simulink model "BMS_Software_NXP_Rolo"  (R2020a)
settings: Solver=FixedStepDiscrete  StartTime=0.0  StopTime=10.0  FixedStep=0.05  RelTol=1e-3  EnableMultiTasking=on
InitFcn:
  | mbd_s32k_consistency_checks(bdroot(gcs));
undefined symbols (not defined in the file or in its folder): LQFP
libraries: mbd_bcc_ec_toolbox x51, mbd_s32k1xx_ec_toolbox x16
(part 1 of 3)
Description:
  | This model demonstrates how to use Model-Based Design Toolbox for S32K to run a BMS Algorithm, already validated in Matlab&Simulink environment.
  | This BMS Algorithm is available for free  on the Mathworks File Exchangehttps://www.mathworks.com/matlabcentral/fileexchange/72865-design-and-test-lithium-ion-battery-management-algorithms
  | 
  | Validation:
  | Hardware required: S32K144EVB + FRDM33772BSPIEVB + BATT-6EMULATOR
  | Once the model has been succesfully build it is automatically deployed on the target.
  | Open the BMS_Software_NXP.pmpx FreeMaster project, connect to the board and simulate the Algorithm states using the Cell Emulator.
settings Model: DataDictionary=BMS_Software_DD_NXP.sldd  EnableAccessToBaseWorkspace=off  PauseTimes=0  ExtModeTrigDuration=5  Creator=Chirag Patel  LastModifiedBy=RolandoA
settings SolverCC: AutoInsertRateTranBlk=on
settings DataIOCC: ExternalInput=off  InitialState=off  SaveOutput=off  SignalLogging=off  SaveTime=off
settings OptimizationCC: DefaultParameterBehavior=Inlined  EnhancedBackFolding=on  PassReuseOutputArgsAs=Individual arguments  ZeroExternalMemoryAtStartup=off  ZeroInternalMemoryAtStartup=off  OptimizeBlockOrder=speed  DifferentSizesBufferReuse=on  OptimizationCustomize=off  EfficientTunableParamExpr=on
settings DebuggingCC: UnderspecifiedInitializationDetection=Classic  MergeDetectMultiDrivingBlocksExec=none  InheritedTsInSrcMsg=none  SingleTaskRateTransMsg=error  ParameterPrecisionLossMsg=none  ParameterTunabilityLossMsg=error  UnconnectedInputMsg=error  UnconnectedOutputMsg=error  UnconnectedLineMsg=error  UnknownTsInhSupMsg=error
settings HardwareCC: ProdBitPerPointer=32  ProdBitPerSizeT=32  ProdBitPerPtrDiffT=32  ProdLargestAtomicInteger=Long  ProdLargestAtomicFloat=Double  ProdWordSize=32  ProdHWDeviceType=ARM Compatible->ARM Cortex
settings ModelReferenceCC: ModelReferenceNumInstancesAllowed=Single  PropagateSignalLabelsOutOfModel=off
settings SFSimCC: MATLABDynamicMemAlloc=off
settings RTWCC: Description=Model Based Design Toolbox S32K1xx Code Generation Target  SystemTargetFile=mbd_s32k.tlc  MakeCommand=mbd_s32k_make_rtw COPY_MDLREF_INCLUDES=0  TemplateMakefile=mbd_s32k.tmf  GenerateReport=on  IncludeHyperlinkInReport=on  LaunchReport=on  GenerateTraceInfo=on  GenerateTraceReport=on  GenerateTraceReportSl=on  GenerateTraceReportSf=on  GenerateTraceReportEml=on
settings CodeAppCC: ForceParamTrailComments=on  IgnoreCustomStorageClasses=off  OperatorAnnotations=on  SimulinkDataObjDesc=on  SFDataObjDesc=on  InsertBlockDesc=on
settings STFCustomTargetCC: TargetLangStandard=C99 (ISO)  MultiwordLength=256  CombineOutputUpdateFcns=on  ERTCustomFileBanners=on  SupportContinuousTime=off  SupportNonInlinedSFcns=off  RemoveResetFunc=on  MATLABClassNameForMDSCustomization=Simulink.SoftwareTarget.ERTCustomization  SystemTargetFile=mbd_s32k.tlc
settings ERTTargetCC: TargetLangStandard=C99 (ISO)  ParMdlRefBuildCompliant=off  CompOptLevelCompliant=off  ConcurrentExecutionCompliant=off  ModelStepFunctionPrototypeControlCompliant=off  CPPClassGenCompliant=off  UseToolchainInfoCompliant=off  InlinedParameterPlacement=NonHierarchical  ERTSrcFileBannerTemplate=mbd_ert_code_template.cgt  ERTHdrFileBannerTemplate=mbd_ert_code_template.cgt  ERTDataSrcFileTemplate=mbd_ert_code_template.cgt  ERTDataHdrFileTemplate=mbd_ert_code_template.cgt  ERTCustomFileTemplate=example_file_process.tlc

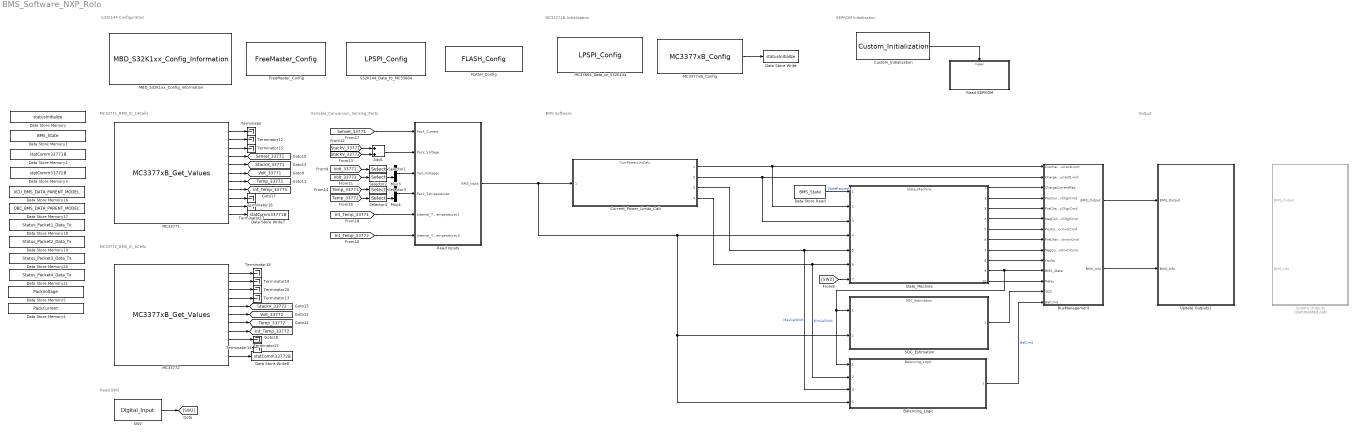
== system BMS_Software_NXP_Rolo ==
  note: EEPROM Initialization
  note: Read SW2
  note: MC33772B Initialization
  note: BMS Software
  note: S32K144 Configuration
  note: Output
  note: MC33771_BMS_IC_14Cells
  note: MC33772_BMS_IC_6Cells
  note: Variable_Conversion_Sensing_Parts
  Add1 : Sum  AccumDataTypeStr=single  OutDataTypeStr=single
  Balancing_Logic : ModelReference  ModelNameDialog=Balancing_Logic  SimulationMode=Normal  ModelReferenceVersion=1.581
      mask Display: image('Balancing.jpg',[70,5,200,90])
  BusManagement : Subsystem
  Current_Power_Limits_Calc : ModelReference  ModelNameDialog=CurrPowerLimCalc.slx  SimulationMode=Normal  ModelReferenceVersion=1.557
      mask Display: image('CurrentPowerLimit.png',[68,15,80,80])
  Custom_Initialization : mbd_s32k1xx_ec_toolbox/Utility Blocks/Custom_Initialization
  Data Store Memory : DataStoreMemory  DataStoreName=statusInitialize  ReadBeforeWriteMsg=warning  WriteAfterWriteMsg=warning  WriteAfterReadMsg=warning  ShowAdditionalParam=off
  Data Store Memory1 : DataStoreMemory  DataStoreName=BMS_State  ReadBeforeWriteMsg=warning  WriteAfterWriteMsg=warning  WriteAfterReadMsg=warning  InitialValue=SRE.Balancing  ShowAdditionalParam=off  OutDataTypeStr=Enum: SRE
  Data Store Memory16 : DataStoreMemory  DataStoreName=VCU_BMS_DATA_PARENT_MODEL  ReadBeforeWriteMsg=warning  WriteAfterWriteMsg=warning  WriteAfterReadMsg=warning  ShowAdditionalParam=off  OutDataTypeStr=Bus: VCU_BMS_DATA
  Data Store Memory17 : DataStoreMemory  DataStoreName=OBC_BMS_DATA_PARENT_MODEL  ReadBeforeWriteMsg=warning  WriteAfterWriteMsg=warning  WriteAfterReadMsg=warning  ShowAdditionalParam=off  OutDataTypeStr=Bus: OBC_BMS_DATA
  Data Store Memory18 : DataStoreMemory  DataStoreName=Status_Packet1_Data_Tx  ReadBeforeWriteMsg=warning  WriteAfterWriteMsg=warning  WriteAfterReadMsg=warning  ShowAdditionalParam=off  OutDataTypeStr=Bus: Status_Packet1_Data_Tx
  Data Store Memory19 : DataStoreMemory  DataStoreName=Status_Packet2_Data_Tx  ReadBeforeWriteMsg=warning  WriteAfterWriteMsg=warning  WriteAfterReadMsg=warning  ShowAdditionalParam=off  OutDataTypeStr=Bus: Status_Packet2_Data_Tx
  Data Store Memory2 : DataStoreMemory  DataStoreName=statComm33771B  ReadBeforeWriteMsg=warning  WriteAfterWriteMsg=warning  WriteAfterReadMsg=warning  ShowAdditionalParam=off
  Data Store Memory20 : DataStoreMemory  DataStoreName=Status_Packet3_Data_Tx  ReadBeforeWriteMsg=warning  WriteAfterWriteMsg=warning  WriteAfterReadMsg=warning  ShowAdditionalParam=off  OutDataTypeStr=Bus: Status_Packet3_Data_Tx
  Data Store Memory21 : DataStoreMemory  DataStoreName=Status_Packet4_Data_Tx  ReadBeforeWriteMsg=warning  WriteAfterWriteMsg=warning  WriteAfterReadMsg=warning  ShowAdditionalParam=off  OutDataTypeStr=Bus: Status_Packet4_Data_Tx
  Data Store Memory3 : DataStoreMemory  DataStoreName=statComm33772B  ReadBeforeWriteMsg=warning  WriteAfterWriteMsg=warning  WriteAfterReadMsg=warning  ShowAdditionalParam=off
  Data Store Memory4 : DataStoreMemory  DataStoreName=PackCurrent  ReadBeforeWriteMsg=warning  WriteAfterWriteMsg=warning  WriteAfterReadMsg=warning  ShowAdditionalParam=off  OutDataTypeStr=single
  Data Store Memory5 : DataStoreMemory  DataStoreName=PackVoltage  ReadBeforeWriteMsg=warning  WriteAfterWriteMsg=warning  WriteAfterReadMsg=warning  ShowAdditionalParam=off  OutDataTypeStr=single
  Data Store Read : DataStoreRead  DataStoreName=BMS_State
  Data Store Write : DataStoreWrite  DataStoreName=statusInitialize
  Data Store Write7 : DataStoreWrite  DataStoreName=statComm33771B
  Data Store Write8 : DataStoreWrite  DataStoreName=statComm33772B
  FLASH_Config : mbd_s32k1xx_ec_toolbox/Core and System Blocks/FLASH Blocks/FLASH_Config  depart=0x2  eeesize=4096  csec_en=off  csec_num_user_keys=5 keys
  FreeMaster_Config : mbd_s32k1xx_ec_toolbox/Utility Blocks/FreeMaster_Config  interface=LPUART2  baudrate=115200  rxd=PTD6: [LPUART2_RX | Receive]  txd=PTD7: [LPUART2_TX | Transmit]  mode=Short Interrupt  isr_prio=1  show_adv_opts=on  use_scope=on  max_scope_vars=8  use_recorder=off  max_rec_vars=8  rec_buff_size=1024  rec_timebase=0 milliseconds  comm_buffer_size_auto=on  comm_buffer_size=255  comm_rqueue_size_default=on  comm_rqueue_size=32
  MBD_S32K1xx_Config_Information : mbd_s32k1xx_ec_toolbox/MBD_S32K1xx_Config_Information  mbdt_ver=0  disp_str=|  config_params=[]  mcu_target_name=S32K144  mcu_target_package=100-LQFP  mcu_target_sram_size=64KB  mcu_system_clock_freq=80  mcu_xtal_freq=External 8  mcu_steptick_timer=LPIT Channel 0  mcu_steptick_prio=15  ds_import_enable=on  target_compiler=GCC  target_memory=FLASH  gcc_target_compile_opts=-mthumb -mfloat-abi=hard -mfpu=fpv4-sp-d16 -O1 -g -gstrict-dwarf  gcc_target_assemble_opts=-mthumb -mfloat-abi=hard -mfpu=fpv4-sp-d16 -g  gcc_target_link_opts=-mthumb -mfloat-abi=hard -mfpu=fpv4-sp-d16  gcc_target_default_lcf=on  gcc_target_user_lcf=S32K148_192_flash.ld  ghs_target_compile_opts=-cpu=cortexm4f -thumb -fpu=vfpv4_d16 -fsingle -Ogeneral -Wundef -Wimplicit-int -Wshadow -Wtrigraphs --no_commons --gnu_asm -gnu99 -gdwarf-2 -G  ghs_target_assemble_opts=-cpu=cortexm4f -fpu=vfpv4_d16  ghs_target_link_opts=-cpu=cortexm4f -thumb -fpu=vfpv4_d16  ghs_target_default_lcf=on  ghs_target_user_lcf=S32K148_192_flash.ld  iar_target_compile_opts=--cpu=Cortex-M4F --thumb --fpu=VFPv4_sp -Ol -e --debug --dlib_config normal  iar_target_assemble_opts=--cpu Cortex-M4F --thumb --fpu VFPv4_sp  iar_target_link_opts=--no_exceptions --vfe --inline  iar_target_default_lcf=on  iar_target_user_lcf=S32K148_192_flash.icf  pil_download_enable=off  rbl_download_enable=on  rbl_start_delay=5000  rbl_download_interface=OpenSDA  rbl_restart_request=off  rbl_com_port=Custom  rbl_com_port_custom=COM1  pil_download_rate=57600  pil_opensda_drive=Custom  pil_opensda_drive_custom=D  pil_uart_instance=1  pil_uart_rx=PTC6: [LPUART1_RX | Receive]  pil_uart_tx=PTC7: [LPUART1_TX | Transmit]  FTM_PWM_PcrCheckEnDis=on  FTM_Input_Edge_Inputs_PcrCheckEnDis=on  FTM_Dual_Edge_Inputs_PcrCheckEnDis=on  FTM_Quadrature_Inputs_PcrCheckEnDis=on  FTM_Hall_Sensor_Inputs_PcrCheckEnDis=on  LPTMR_PcrCheckEnDis=on  PIT_PcrCheckEnDis=on  RTC_PcrCheckEnDis=on  FlexCAN_PcrCheckEnDis=on  LIN_PcrCheckEnDis=on  FlexIO_PcrCheckEnDis=on  LPI2C_PcrCheckEnDis=on  LPSPI_PcrCheckEnDis=on  LPUART_PcrCheckEnDis=on  CMP_PcrCheckEnDis=on  GPIO_OutputPcrCheckEnDis=on  GPIO_InputPcrCheckEnDis=on  SBC_PcrCheckEnDis=on  BMS_PcrCheckEnDis=on  AMMCLIB_PcrCheckEnDis=on  FM_PcrCheckEnDis=on  Profile_PcrCheckEnDis=on  ConfigParams_PcrCheckEnDis=on  ModelRef_PcrCheckEnDis=on  PDB0_PcrCheckEnDis=on  CSEc_PcrCheckEnDis=on  eDMA_PcrCheckEnDis=on  FLASH_PcrCheckEnDis=on  ADC_PcrCheckEnDis=on  WDOG_PcrCheckEnDis=on
      | Target : S32K144-64KB_SRAM
      | Package : 100-pin
      | System clock : 80 MHz
      | XTAL clock : External 8 MHz
      | Compiler : IAR
      | Target Type : FLASH
      | Download Code after build : off
      | Step Tick Interrupt Priority : 15
  MC33664_Data_to_S32K144 : mbd_s32k1xx_ec_toolbox/Communication Blocks/SPI Blocks/LPSPI_Config   InstanceNumber=0  Role=Slave  BaudRate=2000000  ShowAdvanced=on  sin=PTB3: [LPSPI0_SIN | LPSPI Serial Data Input]  sout=PTB4: [LPSPI0_SOUT | LPSPI Serial Data Output]  sck=PTB2: [LPSPI0_SCK | LPSPI Serial Clock I/O]  pcs0=None  pcs1=PTB5: [LPSPI0_PCS1 | Peripheral Chip Select 1]  pcs2=None  pcs3=None  CPHA=1  CPOL=0  BitOrder=MSB first  TransferSize=40  WhichPCS=0  PCSPol=ActiveLow  ContinuousTransfer=off
  MC33771 : mbd_bcc_ec_toolbox/BMS/MC3377xB_Get_Values  bccInstance=0  bccCid=1  bccStartConversion=on
  MC33772 : mbd_bcc_ec_toolbox/BMS/MC3377xB_Get_Values  bccInstance=0  bccCid=2  bccStartConversion=on
  MC3377xB_Config : mbd_bcc_ec_toolbox/BMS/MC3377xB_Config  Priority=1  bccInstance=0  bccMode=TPL  bccTPLDevNr=2  bccSpiDev=MC33772B  bccSpiCell=6  bccTPLDev1=MC33771B  bccTPLCell1=14  bccTPLDev2=MC33772B  bccTPLCell2=6  bccTPLDev3=MC33771B  bccTPLCell3=3  bccTPLDev4=MC33771B  bccTPLCell4=3  bccTPLDev5=MC33771B  bccTPLCell5=3  bccTPLDev6=MC33771B  bccTPLCell6=3  bccTPLDev7=MC33771B  bccTPLCell7=3  bccTPLDev8=MC33771B  bccTPLCell8=3  bccTPLDev9=MC33771B  bccTPLCell9=3  bccTPLDev10=MC33771B  bccTPLCell10=3  bccTPLDev11=MC33771B  bccTPLCell11=3  bccTPLDev12=MC33771B  bccTPLCell12=3  bccTPLDev13=MC33771B  bccTPLCell13=3  bccTPLDev14=MC33771B  bccTPLCell14=3  bccTPLDev15=MC33771B  bccTPLCell15=3  bccSpiMaster=1  bccSPIMasterCSCustom=off  bccSPIMasterPCS=LPSPI_PCS0  bccSPIMasterPCSGPIO=PTA0: [PTA0 | Port A I/O]  bccSpiSlave=0  bccSPISlavePCS=LPSPI_PCS1  bccSPI_RESET_ALT0=PTD4: [PTD4 | Port D I/O]  bccTPL_ENABLE=PTB0: [PTB0 | Port B I/O]  bccTPL_INTB=PTB1: [PTB1 | Port B I/O]  bccNTCBeta=3900  bccNTCRes=6800  bccNTCRefR=10000  bccNTCRefT=25  bccShunt=100000
  Mux3 : Mux  Inputs=2
  Mux4 : Mux  Inputs=2
  Read EEPROM : Subsystem  TreatAsAtomicUnit=on
  Read Inputs : Subsystem
  "S32K144_Data_to_MC33664 " : mbd_s32k1xx_ec_toolbox/Communication Blocks/SPI Blocks/LPSPI_Config   InstanceNumber=1  Role=Master  BaudRate=2000000  ShowAdvanced=on  sin=PTB15: [LPSPI1_SIN | LPSPI Serial Data Input]  sout=PTB16: [LPSPI1_SOUT | LPSPI Serial Data Output]  sck=PTB14: [LPSPI1_SCK | LPSPI Serial Clock I/O]  pcs0=PTD3: [LPSPI1_PCS0 | Peripheral Chip Select 0]  pcs1=None  pcs2=None  pcs3=None  CPHA=1  CPOL=0  BitOrder=MSB first  TransferSize=40  WhichPCS=0  PCSPol=ActiveLow  ContinuousTransfer=off
  SOC_Estimation : ModelReference  ModelNameDialog=SOC_Estimation.slx  SimulationMode=Normal  ModelReferenceVersion=1.802
      mask Display: image('SOC.jpg',[100,15,150,75])
  SW2 : mbd_s32k1xx_ec_toolbox/GPIO Blocks/Digital_Input  gpio_pin=PTC12: [PTC12 | Port C I/O]  pull_resistor=Pulldown  passive_filter=off
  Selector1 : Selector  InputPortWidth=14  IndexOptions=Index vector (dialog)  Indices=[1:14]  OutputSizes=1
  Selector2 : Selector  InputPortWidth=14  IndexOptions=Index vector (dialog)  Indices=[1:6]  OutputSizes=1
  Selector3 : Selector  InputPortWidth=7  IndexOptions=Index vector (dialog)  Indices=[1:7]  OutputSizes=1
  Selector4 : Selector  InputPortWidth=7  IndexOptions=Index vector (dialog)  Indices=[1:7]  OutputSizes=1
  State_Machine : ModelReference  ModelNameDialog=State_Machine  SimulationMode=Normal  ModelReferenceVersion=1.745
      mask Display: image('StateMachine.jpg',[80,40,130,130])
  Terminator{,12..21} (11 alike) : Terminator
  Update Outputs : Subsystem  Commented=on
  Update Outputs1 : Subsystem
  tag scope: Int_Temp_33771=global, Int_Temp_33772=global, SenseI_33771=global, StackV_33771=global, StackV_33772=global, Temp_33771=global, Temp_33772=global, Volt_33771=global, Volt_33772=global
  wires:
  Data Store Read/1 -> State_Machine/1  "StateRequest"
  MC3377xB_Config/1 -> Data Store Write/1
  BusManagement/1(BMS_Output) -> Update Outputs1/1(BMS_Output)
  BusManagement/2(BMS_Info) -> Update Outputs1/2(BMS_Info)
  Current_Power_Limits_Calc/3 -> Balancing_Logic/3, State_Machine/5  "MaxCellVolt"
  Current_Power_Limits_Calc/4 -> Balancing_Logic/2, State_Machine/6  "MinCellVolt"
  SW2/1 -> [SW2]
  [SW2] -> State_Machine/7
  Current_Power_Limits_Calc/2 -> State_Machine/3, BusManagement/2(ChargeCurrentLimit)
  Current_Power_Limits_Calc/1 -> State_Machine/2, BusManagement/1(DischargeCurrentLimit)
  State_Machine/1 -> BusManagement/3(ChargeCurrentReq)
  State_Machine/2 -> BusManagement/4(PosContactorChgrCmd)
  State_Machine/8 -> BusManagement/10(Faults)
  State_Machine/7 -> BusManagement/9(NegContactorInvtrCmd)
  State_Machine/6 -> BusManagement/8(PreChargeRelayInvtrCmd)
  State_Machine/5 -> BusManagement/7(PosContactorInvtrCmd)
  State_Machine/4 -> BusManagement/6(NegContactorChgrCmd)
  State_Machine/3 -> BusManagement/5(PreChargeRelayChgrCmd)
  State_Machine/9 -> BusManagement/11(BMS_State), Balancing_Logic/1, SOC_Estimation/1
  State_Machine/10 -> BusManagement/12(Relay)
  SOC_Estimation/1 -> BusManagement/13(SOC)
  Balancing_Logic/1 -> BusManagement/14(BalCmd)  "BalCmd"
  MC33771/2 -> Terminator12/1
  Selector2/1 -> Mux3/2
  MC33772/1 -> Terminator18/1
  MC33772/10 -> Terminator14/1
  Selector1/1 -> Mux3/1
  MC33771/10 -> Terminator17/1
  MC33771/9 -> Terminator16/1
  MC33772/2 -> Terminator19/1
  MC33771/4 -> [SenseI_33771]
  [Int_Temp_33772] -> Read Inputs/6(Internal_Temperaturev2)
  Selector4/1 -> Mux4/2
  [Volt_33771] -> Selector1/1
  [StackV_33771] -> Add1/1
  [SenseI_33771] -> Read Inputs/1(Pack_Current)
  MC33772/9 -> Terminator21/1
  [Temp_33772] -> Selector4/1
  MC33771/6 -> [Volt_33771]
  [Temp_33771] -> Selector3/1
  MC33771/8 -> [Int_Temp_33771]
  Selector3/1 -> Mux4/1
  MC33772/4 -> Terminator13/1
  [Volt_33772] -> Selector2/1
  MC33772/6 -> [Volt_33772]
  MC33771/7 -> [Temp_33771]
  MC33772/3 -> Terminator20/1
  MC33771/1 -> Terminator/1
  Add1/1 -> Read Inputs/2(Pack_Voltage)
  MC33772/5 -> [StackV_33772]
  MC33771/5 -> [StackV_33771]
  MC33772/7 -> [Temp_33772]
  [Int_Temp_33771] -> Read Inputs/5(Internal_Temperaturev1)
  MC33771/3 -> Terminator15/1
  MC33772/8 -> [Int_Temp_33772]
  [StackV_33772] -> Add1/2
  Read Inputs/1(BMS_Input) -> Balancing_Logic/4, SOC_Estimation/2, State_Machine/4, Current_Power_Limits_Calc/1
  Mux3/1 -> Read Inputs/3(Cell_Voltages)
  Mux4/1 -> Read Inputs/4(Pack_Temperatures)
  MC33772/11 -> Data Store Write8/1
  MC33771/11 -> Data Store Write7/1
  Custom_Initialization/1 -> Read EEPROM/Trigger

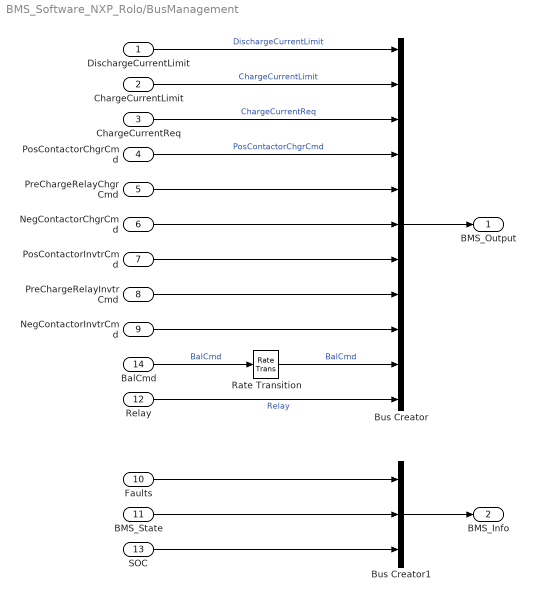
== system BMS_Software_NXP_Rolo/BusManagement ==
  DischargeCurrentLimit : Inport
  ChargeCurrentLimit : Inport  Port=2
  ChargeCurrentReq : Inport  Port=3
  PosContactorChgrCmd : Inport  Port=4
  PreChargeRelayChgrCmd : Inport  Port=5
  NegContactorChgrCmd : Inport  Port=6
  PosContactorInvtrCmd : Inport  Port=7
  PreChargeRelayInvtrCmd : Inport  Port=8
  NegContactorInvtrCmd : Inport  Port=9
  Faults : Inport  Port=10
  BMS_State : Inport  Port=11
  Relay : Inport  Port=12
  SOC : Inport  Port=13
  BalCmd : Inport  Port=14
  Bus Creator1 : BusCreator  Inputs=3  OutDataTypeStr=Bus: BMS_Info  NonVirtualBus=on
  Bus Creator : BusCreator  Inputs=11  OutDataTypeStr=Bus: BMS_Output  NonVirtualBus=on
  Rate Transition : RateTransition  Integrity=off  Deterministic=off
  BMS_Output : Outport
  BMS_Info : Outport  Port=2  OutDataTypeStr=Bus: BMS_Info
  wires:
  PosContactorInvtrCmd/1 -> Bus Creator/7
  PreChargeRelayChgrCmd/1 -> Bus Creator/5
  PosContactorChgrCmd/1 -> Bus Creator/4  "PosContactorChgrCmd"
  NegContactorInvtrCmd/1 -> Bus Creator/9
  Faults/1 -> Bus Creator1/1
  NegContactorChgrCmd/1 -> Bus Creator/6
  PreChargeRelayInvtrCmd/1 -> Bus Creator/8
  Bus Creator1/1 -> BMS_Info/1
  Bus Creator/1 -> BMS_Output/1
  SOC/1 -> Bus Creator1/3
  BMS_State/1 -> Bus Creator1/2
  ChargeCurrentLimit/1 -> Bus Creator/2  "ChargeCurrentLimit"
  DischargeCurrentLimit/1 -> Bus Creator/1  "DischargeCurrentLimit"
  ChargeCurrentReq/1 -> Bus Creator/3  "ChargeCurrentReq"
  BalCmd/1 -> Rate Transition/1  "BalCmd"
  Rate Transition/1 -> Bus Creator/10  "BalCmd"
  Relay/1 -> Bus Creator/11  "Relay"

== system BMS_Software_NXP_Rolo/Read EEPROM ==
  function : TriggerPort  TriggerType=function-call  VariantControl=Variant
  Data Store Write1 : DataStoreWrite  DataStoreName=PreviousSOC
  Data Store Write2 : DataStoreWrite  DataStoreName=LockOCVTable
  FLASH_EEERead : mbd_s32k1xx_ec_toolbox/Core and System Blocks/FLASH Blocks/FLASH_EEERead  base=0x14000000  offset=0x0000  ptr=uint8_t
  FLASH_EEERead1 : mbd_s32k1xx_ec_toolbox/Core and System Blocks/FLASH Blocks/FLASH_EEERead  base=0x14000000  offset=0x0001  ptr=uint8_t
  wires:
  FLASH_EEERead/1 -> Data Store Write1/1
  FLASH_EEERead1/1 -> Data Store Write2/1

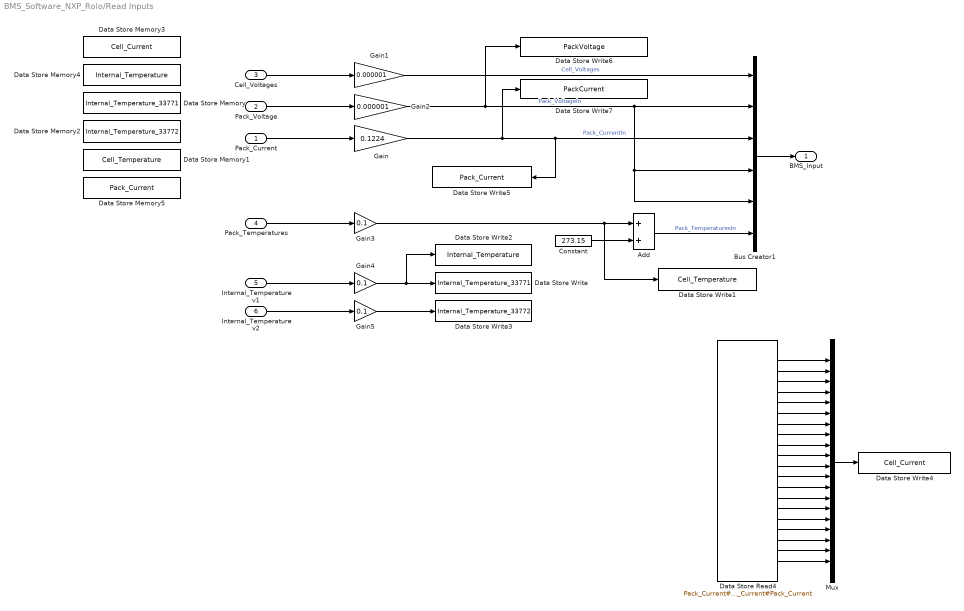
== system BMS_Software_NXP_Rolo/Read Inputs ==
  Pack_Current : Inport
  Pack_Voltage : Inport  Port=2
  Cell_Voltages : Inport  Port=3
  Pack_Temperatures : Inport  Port=4
  Internal_Temperaturev1 : Inport  Port=5
  Internal_Temperaturev2 : Inport  Port=6
  Add : Sum  OutDataTypeStr=single
  Bus Creator1 : BusCreator  Inputs=6  OutDataTypeStr=Bus: BMS_Input  NonVirtualBus=on
      settings: InheritFromInputs=off
  Constant : Constant  Value=273.15  OutDataTypeStr=single
  Data Store Memory : DataStoreMemory  DataStoreName=Internal_Temperature_33771  ReadBeforeWriteMsg=warning  WriteAfterWriteMsg=warning  WriteAfterReadMsg=warning  ShowAdditionalParam=off  OutDataTypeStr=single
  Data Store Memory1 : DataStoreMemory  DataStoreName=Cell_Temperature  ReadBeforeWriteMsg=warning  WriteAfterWriteMsg=warning  WriteAfterReadMsg=warning  InitialValue=[ 0 0 0 0 0 0 0 0 0 0 0 0 0 0]  ShowAdditionalParam=off  OutDataTypeStr=single
  Data Store Memory2 : DataStoreMemory  DataStoreName=Internal_Temperature_33772  ReadBeforeWriteMsg=warning  WriteAfterWriteMsg=warning  WriteAfterReadMsg=warning  ShowAdditionalParam=off  OutDataTypeStr=single
  Data Store Memory3 : DataStoreMemory  DataStoreName=Cell_Current  ReadBeforeWriteMsg=warning  WriteAfterWriteMsg=warning  WriteAfterReadMsg=warning  InitialValue=[ 0 0 0 0 0 0 0 0 0 0 0 0 0 0 0 0 0 0 0 0]  ShowAdditionalParam=off  OutDataTypeStr=single
  Data Store Memory4 : DataStoreMemory  DataStoreName=Internal_Temperature  ReadBeforeWriteMsg=warning  WriteAfterWriteMsg=warning  WriteAfterReadMsg=warning  ShowAdditionalParam=off  OutDataTypeStr=single
  Data Store Memory5 : DataStoreMemory  DataStoreName=Pack_Current  ReadBeforeWriteMsg=warning  WriteAfterWriteMsg=warning  WriteAfterReadMsg=warning  ShowAdditionalParam=off  OutDataTypeStr=single
  Data Store Read4 : DataStoreRead  DataStoreName=Pack_Current  DataStoreElements=Pack_Current#Pack_Current#Pack_Current#Pack_Current#Pack_Current#Pack_Current#Pack_Current#Pack_Current#Pack_Current#Pack_Current#Pack_Current#Pack_Current#Pack_Current#Pack_Current#Pack_Current#Pack_Current#Pack_Current#Pack_Current#Pack_Current#Pack_Current
  Data Store Write : DataStoreWrite  DataStoreName=Internal_Temperature_33771
  Data Store Write1 : DataStoreWrite  DataStoreName=Cell_Temperature
  Data Store Write2 : DataStoreWrite  DataStoreName=Internal_Temperature
  Data Store Write3 : DataStoreWrite  DataStoreName=Internal_Temperature_33772
  Data Store Write4 : DataStoreWrite  DataStoreName=Cell_Current
  Data Store Write5 : DataStoreWrite  DataStoreName=Pack_Current
  Data Store Write6 : DataStoreWrite  DataStoreName=PackVoltage
  Data Store Write7 : DataStoreWrite  DataStoreName=PackCurrent
  Gain : Gain  Gain=0.1224  OutDataTypeStr=Inherit: Inherit via back propagation
  Gain1 : Gain  Gain=0.000001  OutDataTypeStr=Inherit: Inherit via back propagation
  Gain2 : Gain  Gain=0.000001  OutDataTypeStr=Inherit: Inherit via back propagation
  Gain3 : Gain  Gain=0.1  OutDataTypeStr=single
  Gain4 : Gain  Gain=0.1  OutDataTypeStr=single
  Gain5 : Gain  Gain=0.1  OutDataTypeStr=single
  Mux : Mux  Inputs=20
  BMS_Input : Outport
  wires:
  Bus Creator1/1 -> BMS_Input/1
  Pack_Voltage/1 -> Gain2/1
  Pack_Current/1 -> Gain/1
  Gain/1 -> Data Store Write7/1, Data Store Write5/1, Bus Creator1/3  "Pack_CurrentIn"
  Gain2/1 -> Data Store Write6/1, Bus Creator1/2, Bus Creator1/4, Bus Creator1/5  "Pack_VoltageIn"
  Constant/1 -> Add/2
  Gain3/1 -> Data Store Write1/1, Add/1
  Internal_Temperaturev1/1 -> Gain4/1
  Gain4/1 -> Data Store Write2/1, Data Store Write/1
  Cell_Voltages/1 -> Gain1/1
  Gain1/1 -> Bus Creator1/1  "Cell_Voltages"
  Gain5/1 -> Data Store Write3/1
  Internal_Temperaturev2/1 -> Gain5/1
  Pack_Temperatures/1 -> Gain3/1
  Mux/1 -> Data Store Write4/1
  Data Store Read4/1 -> Mux/1
  Data Store Read4/2 -> Mux/2
  Data Store Read4/3 -> Mux/3
  Data Store Read4/4 -> Mux/4
  Data Store Read4/5 -> Mux/5
  Data Store Read4/6 -> Mux/6
  Data Store Read4/7 -> Mux/7
  Data Store Read4/8 -> Mux/8
  Data Store Read4/9 -> Mux/9
  Data Store Read4/10 -> Mux/10
  Data Store Read4/11 -> Mux/11
  Data Store Read4/12 -> Mux/12
  Data Store Read4/13 -> Mux/13
  Data Store Read4/14 -> Mux/14
  Data Store Read4/15 -> Mux/15
  Data Store Read4/16 -> Mux/16
  Data Store Read4/17 -> Mux/17
  Data Store Read4/18 -> Mux/18
  Data Store Read4/19 -> Mux/19
  Data Store Read4/20 -> Mux/20
  Add/1 -> Bus Creator1/6  "Pack_TemperaturesIn"

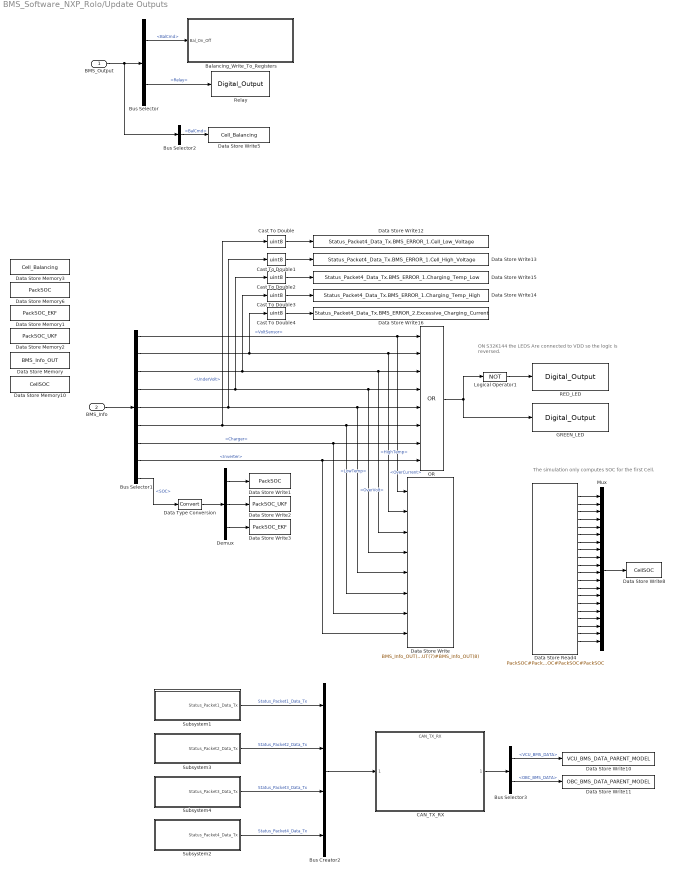
== system BMS_Software_NXP_Rolo/Update Outputs ==
  note: ON S32K144 the LEDS Are connected to VDD so the logic is reversed.
  note: The simulation only computes SOC for the first Cell.
  BMS_Output : Inport
  BMS_Info : Inport  Port=2
  Balancing_Write_To_Registers : Subsystem
  Bus Creator2 : BusCreator  Inputs=4  OutDataTypeStr=Bus: ALL_TX_DATA  NonVirtualBus=on
  Bus Selector : BusSelector  OutputSignals=BalCmd,Relay
  Bus Selector1 : BusSelector  OutputSignals=Faults.VoltSensor,Faults.OverCurrent,Faults.HighTemp,Faults.LowTemp,Faults.OverVolt,Faults.UnderVolt,Faults.Charger,Faults.Inverter,SOC
  Bus Selector2 : BusSelector  OutputSignals=BalCmd
  Bus Selector3 : BusSelector  OutputSignals=VCU_BMS_DATA,OBC_BMS_DATA
  CAN_TX_RX : ModelReference  ModelNameDialog=CAN_TX_RX.slx  SimulationMode=Normal  ModelReferenceVersion=1.147
  Cast To Double{,1..4} (5 alike) : DataTypeConversion  OutDataTypeStr=uint8
  Data Store Memory : DataStoreMemory  DataStoreName=BMS_Info_OUT  ReadBeforeWriteMsg=warning  WriteAfterWriteMsg=warning  WriteAfterReadMsg=warning  InitialValue=[0 0 0 0 0 0 0 0]  ShowAdditionalParam=off  OutDataTypeStr=boolean
  Data Store Memory1 : DataStoreMemory  DataStoreName=PackSOC_EKF  ReadBeforeWriteMsg=warning  WriteAfterWriteMsg=warning  WriteAfterReadMsg=warning  ShowAdditionalParam=off  OutDataTypeStr=single
  Data Store Memory10 : DataStoreMemory  DataStoreName=CellSOC  ReadBeforeWriteMsg=warning  WriteAfterWriteMsg=warning  WriteAfterReadMsg=warning  InitialValue=zeros(1,20)  ShowAdditionalParam=off  OutDataTypeStr=single
  Data Store Memory2 : DataStoreMemory  DataStoreName=PackSOC_UKF  ReadBeforeWriteMsg=warning  WriteAfterWriteMsg=warning  WriteAfterReadMsg=warning  ShowAdditionalParam=off  OutDataTypeStr=single
  Data Store Memory3 : DataStoreMemory  DataStoreName=Cell_Balancing  ReadBeforeWriteMsg=warning  WriteAfterWriteMsg=warning  WriteAfterReadMsg=warning  InitialValue=[0 0 0 0 0 0 0 0 0 0 0 0 0 0 0 0 0 0 0 0]  ShowAdditionalParam=off  OutDataTypeStr=boolean
  Data Store Memory6 : DataStoreMemory  DataStoreName=PackSOC  ReadBeforeWriteMsg=warning  WriteAfterWriteMsg=warning  WriteAfterReadMsg=warning  ShowAdditionalParam=off  OutDataTypeStr=single
  Data Store Read4 : DataStoreRead  DataStoreName=PackSOC  DataStoreElements=PackSOC#PackSOC#PackSOC#PackSOC#PackSOC#PackSOC#PackSOC#PackSOC#PackSOC#PackSOC#PackSOC#PackSOC#PackSOC#PackSOC#PackSOC#PackSOC#PackSOC#PackSOC#PackSOC#PackSOC
  Data Store Write : DataStoreWrite  DataStoreName=BMS_Info_OUT  DataStoreElements=BMS_Info_OUT(1)#BMS_Info_OUT(2)#BMS_Info_OUT(3)#BMS_Info_OUT(4)#BMS_Info_OUT(5)#BMS_Info_OUT(6)#BMS_Info_OUT(7)#BMS_Info_OUT(8)
  Data Store Write1 : DataStoreWrite  DataStoreName=PackSOC
  Data Store Write10 : DataStoreWrite  DataStoreName=VCU_BMS_DATA_PARENT_MODEL
  Data Store Write11 : DataStoreWrite  DataStoreName=OBC_BMS_DATA_PARENT_MODEL
  Data Store Write12 : DataStoreWrite  DataStoreName=Status_Packet4_Data_Tx  DataStoreElements=Status_Packet4_Data_Tx.BMS_ERROR_1.Cell_Low_Voltage
  Data Store Write13 : DataStoreWrite  DataStoreName=Status_Packet4_Data_Tx  DataStoreElements=Status_Packet4_Data_Tx.BMS_ERROR_1.Cell_High_Voltage
  Data Store Write14 : DataStoreWrite  DataStoreName=Status_Packet4_Data_Tx  DataStoreElements=Status_Packet4_Data_Tx.BMS_ERROR_1.Charging_Temp_High
  Data Store Write15 : DataStoreWrite  DataStoreName=Status_Packet4_Data_Tx  DataStoreElements=Status_Packet4_Data_Tx.BMS_ERROR_1.Charging_Temp_Low
  Data Store Write16 : DataStoreWrite  DataStoreName=Status_Packet4_Data_Tx  DataStoreElements=Status_Packet4_Data_Tx.BMS_ERROR_2.Excessive_Charging_Current
  Data Store Write2 : DataStoreWrite  DataStoreName=PackSOC_UKF
  Data Store Write3 : DataStoreWrite  DataStoreName=PackSOC_EKF
  Data Store Write5 : DataStoreWrite  DataStoreName=Cell_Balancing
  Data Store Write8 : DataStoreWrite  DataStoreName=CellSOC
  Data Type Conversion : DataTypeConversion
  Demux : Demux  Outputs=3
  GREEN_LED : mbd_s32k1xx_ec_toolbox/GPIO Blocks/Digital_Output  gpio_pin=PTD16: [PTD16 | Port D I/O]  init_val=Low  drive_strength=Low
  Logical Operator1 : Logic  Operator=NOT  AllPortsSameDT=off  OutDataTypeStr=boolean
  Mux : Mux  Inputs=20
  OR : Logic  Operator=OR  Inputs=8  AllPortsSameDT=off  OutDataTypeStr=boolean
  RED_LED : mbd_s32k1xx_ec_toolbox/GPIO Blocks/Digital_Output  gpio_pin=PTD15: [PTD15 | Port D I/O]  init_val=Low  drive_strength=Low
  Relay : mbd_s32k1xx_ec_toolbox/GPIO Blocks/Digital_Output  gpio_pin=PTD10: [PTD10 | Port D I/O]  init_val=Low  drive_strength=High
  Subsystem1 : Subsystem
  Subsystem2 : Subsystem
  Subsystem3 : Subsystem
  Subsystem4 : Subsystem
  wires:
  Bus Selector1/4 -> Cast To Double2/1, OR/4, Data Store Write/4  "<LowTemp>"
  Bus Selector1/8 -> OR/8, Data Store Write/8  "<Inverter>"
  OR/1 -> Logical Operator1/1, GREEN_LED/1
  Bus Selector1/5 -> Cast To Double1/1, OR/5, Data Store Write/5  "<OverVolt>"
  Bus Selector1/7 -> OR/7, Data Store Write/7  "<Charger>"
  Bus Selector1/3 -> Cast To Double3/1, OR/3, Data Store Write/3  "<HighTemp>"
  Bus Selector1/1 -> OR/1, Data Store Write/1  "<VoltSensor>"
  Bus Selector1/6 -> Cast To Double/1, OR/6, Data Store Write/6  "<UnderVolt>"
  Bus Selector1/2 -> Cast To Double4/1, OR/2, Data Store Write/2  "<OverCurrent>"
  BMS_Info/1 -> Bus Selector1/1
  Logical Operator1/1 -> RED_LED/1
  Bus Selector1/9 -> Data Type Conversion/1  "<SOC>"
  Data Type Conversion/1 -> Demux/1
  Demux/1 -> Data Store Write1/1
  Demux/2 -> Data Store Write2/1
  Demux/3 -> Data Store Write3/1
  Data Store Read4/1 -> Mux/1
  Data Store Read4/2 -> Mux/2
  Data Store Read4/3 -> Mux/3
  Data Store Read4/4 -> Mux/4
  Data Store Read4/5 -> Mux/5
  Data Store Read4/6 -> Mux/6
  Data Store Read4/7 -> Mux/7
  Data Store Read4/8 -> Mux/8
  Data Store Read4/9 -> Mux/9
  Data Store Read4/10 -> Mux/10
  Data Store Read4/11 -> Mux/11
  Data Store Read4/12 -> Mux/12
  Data Store Read4/13 -> Mux/13
  Data Store Read4/14 -> Mux/14
  Data Store Read4/15 -> Mux/15
  Data Store Read4/16 -> Mux/16
  Data Store Read4/17 -> Mux/17
  Data Store Read4/18 -> Mux/18
  Data Store Read4/19 -> Mux/19
  Data Store Read4/20 -> Mux/20
  Mux/1 -> Data Store Write8/1
  BMS_Output/1 -> Bus Selector2/1, Bus Selector/1
  Bus Selector/1 -> Balancing_Write_To_Registers/1(Bal_On_Off)  "<BalCmd>"
  Bus Creator2/1 -> CAN_TX_RX/1
  Subsystem1/1(Status_Packet1_Data_Tx) -> Bus Creator2/1  "Status_Packet1_Data_Tx"
  Subsystem3/1(Status_Packet2_Data_Tx) -> Bus Creator2/2  "Status_Packet2_Data_Tx"
  Subsystem2/1(Status_Packet4_Data_Tx) -> Bus Creator2/4  "Status_Packet4_Data_Tx"
  Subsystem4/1(Status_Packet3_Data_Tx) -> Bus Creator2/3  "Status_Packet3_Data_Tx"
  Cast To Double/1 -> Data Store Write12/1
  Cast To Double1/1 -> Data Store Write13/1
  Cast To Double2/1 -> Data Store Write15/1
  Cast To Double3/1 -> Data Store Write14/1
  Cast To Double4/1 -> Data Store Write16/1
  Bus Selector3/1 -> Data Store Write10/1  "<VCU_BMS_DATA>"
  Bus Selector3/2 -> Data Store Write11/1  "<OBC_BMS_DATA>"
  CAN_TX_RX/1 -> Bus Selector3/1
  Bus Selector/2 -> Relay/1  "<Relay>"
  Bus Selector2/1 -> Data Store Write5/1  "<BalCmd>"

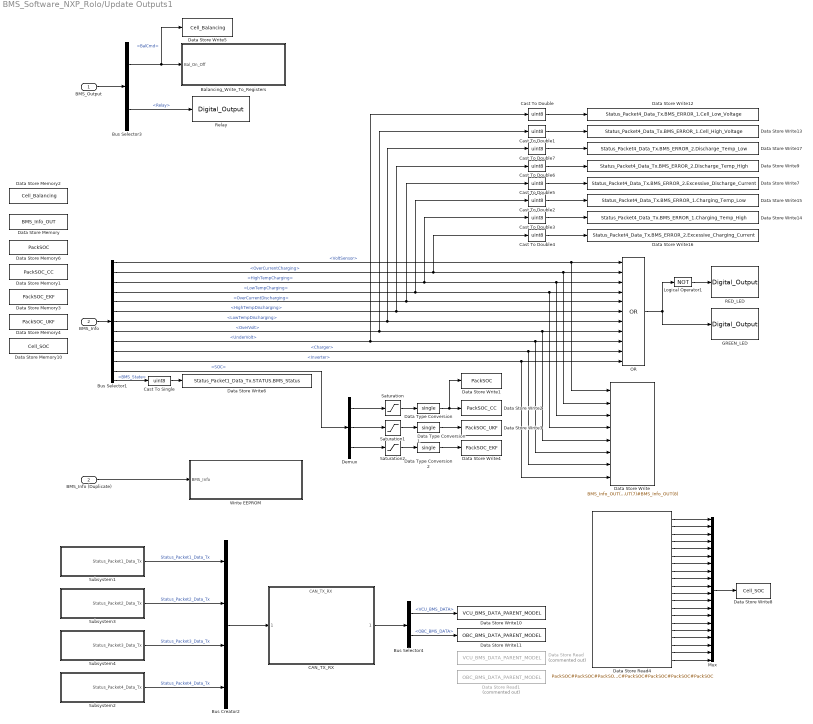
== system BMS_Software_NXP_Rolo/Update Outputs1 ==
  BMS_Output : Inport
  BMS_Info : Inport  Port=2
  BMS_Info (Duplicate) : InportShadow  Port=2
  Balancing_Write_To_Registers : Subsystem
  Bus Creator2 : BusCreator  Inputs=4  OutDataTypeStr=Bus: ALL_TX_DATA  NonVirtualBus=on
  Bus Selector1 : BusSelector  OutputSignals=Faults.VoltSensor,Faults.OverCurrentCharging,Faults.HighTempCharging,Faults.LowTempCharging,Faults.OverCurrentDischarging,Faults.HighTempDischarging,Faults.LowTempDischarging,Faults.OverVolt,Faults.UnderVolt,Faults.Charger,Faults.Inverter,SOC,BMS_State
  Bus Selector3 : BusSelector  OutputSignals=BalCmd,Relay
  Bus Selector4 : BusSelector  OutputSignals=VCU_BMS_DATA,OBC_BMS_DATA
  CAN_TX_RX : ModelReference  ModelNameDialog=CAN_TX_RX.slx  SimulationMode=Normal  ModelReferenceVersion=1.148
  Cast To Double{,1..7} (8 alike) : DataTypeConversion  OutDataTypeStr=uint8
  Cast To Single : DataTypeConversion  OutDataTypeStr=uint8
  Data Store Memory : DataStoreMemory  DataStoreName=BMS_Info_OUT  ReadBeforeWriteMsg=warning  WriteAfterWriteMsg=warning  WriteAfterReadMsg=warning  InitialValue=[0 0 0 0 0 0 0 0]  ShowAdditionalParam=off  OutDataTypeStr=boolean
  Data Store Memory1 : DataStoreMemory  DataStoreName=PackSOC_CC  ReadBeforeWriteMsg=warning  WriteAfterWriteMsg=warning  WriteAfterReadMsg=warning  ShowAdditionalParam=off  OutDataTypeStr=single
  Data Store Memory10 : DataStoreMemory  DataStoreName=Cell_SOC  ReadBeforeWriteMsg=warning  WriteAfterWriteMsg=warning  WriteAfterReadMsg=warning  InitialValue=zeros(1,20)  ShowAdditionalParam=off  OutDataTypeStr=single
  Data Store Memory2 : DataStoreMemory  DataStoreName=Cell_Balancing  ReadBeforeWriteMsg=warning  WriteAfterWriteMsg=warning  WriteAfterReadMsg=warning  InitialValue=[0 0 0 0 0 0 0 0 0 0 0 0 0 0 0 0 0 0 0 0]  ShowAdditionalParam=off  OutDataTypeStr=boolean
  Data Store Memory3 : DataStoreMemory  DataStoreName=PackSOC_EKF  ReadBeforeWriteMsg=warning  WriteAfterWriteMsg=warning  WriteAfterReadMsg=warning  ShowAdditionalParam=off  OutDataTypeStr=single
  Data Store Memory4 : DataStoreMemory  DataStoreName=PackSOC_UKF  ReadBeforeWriteMsg=warning  WriteAfterWriteMsg=warning  WriteAfterReadMsg=warning  ShowAdditionalParam=off  OutDataTypeStr=single
  Data Store Memory6 : DataStoreMemory  DataStoreName=PackSOC  ReadBeforeWriteMsg=warning  WriteAfterWriteMsg=warning  WriteAfterReadMsg=warning  ShowAdditionalParam=off  OutDataTypeStr=single
  Data Store Read : DataStoreRead  Commented=on  DataStoreName=VCU_BMS_DATA_PARENT_MODEL
  Data Store Read1 : DataStoreRead  Commented=on  DataStoreName=OBC_BMS_DATA_PARENT_MODEL
  Data Store Read4 : DataStoreRead  DataStoreName=PackSOC  DataStoreElements=PackSOC#PackSOC#PackSOC#PackSOC#PackSOC#PackSOC#PackSOC#PackSOC#PackSOC#PackSOC#PackSOC#PackSOC#PackSOC#PackSOC#PackSOC#PackSOC#PackSOC#PackSOC#PackSOC#PackSOC
  Data Store Write : DataStoreWrite  DataStoreName=BMS_Info_OUT  DataStoreElements=BMS_Info_OUT(1)#BMS_Info_OUT(2)#BMS_Info_OUT(3)#BMS_Info_OUT(4)#BMS_Info_OUT(5)#BMS_Info_OUT(6)#BMS_Info_OUT(7)#BMS_Info_OUT(8)
  Data Store Write1 : DataStoreWrite  DataStoreName=PackSOC
  Data Store Write10 : DataStoreWrite  DataStoreName=VCU_BMS_DATA_PARENT_MODEL
  Data Store Write11 : DataStoreWrite  DataStoreName=OBC_BMS_DATA_PARENT_MODEL
  Data Store Write12 : DataStoreWrite  DataStoreName=Status_Packet4_Data_Tx  DataStoreElements=Status_Packet4_Data_Tx.BMS_ERROR_1.Cell_Low_Voltage
  Data Store Write13 : DataStoreWrite  DataStoreName=Status_Packet4_Data_Tx  DataStoreElements=Status_Packet4_Data_Tx.BMS_ERROR_1.Cell_High_Voltage
  Data Store Write14 : DataStoreWrite  DataStoreName=Status_Packet4_Data_Tx  DataStoreElements=Status_Packet4_Data_Tx.BMS_ERROR_1.Charging_Temp_High
  Data Store Write15 : DataStoreWrite  DataStoreName=Status_Packet4_Data_Tx  DataStoreElements=Status_Packet4_Data_Tx.BMS_ERROR_1.Charging_Temp_Low
  Data Store Write16 : DataStoreWrite  DataStoreName=Status_Packet4_Data_Tx  DataStoreElements=Status_Packet4_Data_Tx.BMS_ERROR_2.Excessive_Charging_Current
  Data Store Write17 : DataStoreWrite  DataStoreName=Status_Packet4_Data_Tx  DataStoreElements=Status_Packet4_Data_Tx.BMS_ERROR_2.Discharge_Temp_Low
  Data Store Write2 : DataStoreWrite  DataStoreName=PackSOC_CC
  Data Store Write3 : DataStoreWrite  DataStoreName=PackSOC_UKF
  Data Store Write4 : DataStoreWrite  DataStoreName=PackSOC_EKF
  Data Store Write5 : DataStoreWrite  DataStoreName=Cell_Balancing
  Data Store Write6 : DataStoreWrite  DataStoreName=Status_Packet1_Data_Tx  DataStoreElements=Status_Packet1_Data_Tx.STATUS.BMS_Status
  Data Store Write7 : DataStoreWrite  DataStoreName=Status_Packet4_Data_Tx  DataStoreElements=Status_Packet4_Data_Tx.BMS_ERROR_2.Excessive_Discharge_Current
  Data Store Write8 : DataStoreWrite  DataStoreName=Cell_SOC
  Data Store Write9 : DataStoreWrite  DataStoreName=Status_Packet4_Data_Tx  DataStoreElements=Status_Packet4_Data_Tx.BMS_ERROR_2.Discharge_Temp_High
  Data Type Conversion : DataTypeConversion  OutDataTypeStr=single
  Data Type Conversion1 : DataTypeConversion  OutDataTypeStr=single
  Data Type Conversion2 : DataTypeConversion  OutDataTypeStr=single
  Demux : Demux  Outputs=3
  GREEN_LED : mbd_s32k1xx_ec_toolbox/GPIO Blocks/Digital_Output  gpio_pin=PTD16: [PTD16 | Port D I/O]  init_val=Low  drive_strength=Low
  Logical Operator1 : Logic  Operator=NOT  AllPortsSameDT=off  OutDataTypeStr=boolean
  Mux : Mux  Inputs=20
  OR : Logic  Operator=OR  Inputs=11  AllPortsSameDT=off  OutDataTypeStr=boolean
  RED_LED : mbd_s32k1xx_ec_toolbox/GPIO Blocks/Digital_Output  gpio_pin=PTD15: [PTD15 | Port D I/O]  init_val=Low  drive_strength=Low
  Relay : mbd_s32k1xx_ec_toolbox/GPIO Blocks/Digital_Output  gpio_pin=PTD10: [PTD10 | Port D I/O]  init_val=Low  drive_strength=High
  Saturation : Saturate  UpperLimit=1  LowerLimit=0
  Saturation1 : Saturate  UpperLimit=1  LowerLimit=0
  Saturation2 : Saturate  UpperLimit=1  LowerLimit=0
  Subsystem1 : Subsystem
  Subsystem2 : Subsystem
  Subsystem3 : Subsystem
  Subsystem4 : Subsystem
  Write EEPROM : Subsystem
  wires:
  OR/1 -> Logical Operator1/1, GREEN_LED/1
  Bus Selector1/1 -> Data Store Write/1, OR/1  "<VoltSensor>"
  BMS_Info/1 -> Bus Selector1/1
  Data Store Read4/6 -> Mux/6
  Mux/1 -> Data Store Write8/1
  Data Store Read4/1 -> Mux/1
  Data Store Read4/4 -> Mux/4
  Data Store Read4/5 -> Mux/5
  Data Store Read4/3 -> Mux/3
  Demux/1 -> Saturation/1
  Data Store Read4/2 -> Mux/2
  Demux/2 -> Saturation1/1
  Demux/3 -> Saturation2/1
  Data Type Conversion/1 -> Data Store Write1/1, Data Store Write2/1
  Data Type Conversion1/1 -> Data Store Write3/1
  Data Type Conversion2/1 -> Data Store Write4/1
  Saturation/1 -> Data Type Conversion/1
  Data Store Read4/7 -> Mux/7
  Data Store Read4/8 -> Mux/8
  Data Store Read4/9 -> Mux/9
  Data Store Read4/10 -> Mux/10
  Data Store Read4/11 -> Mux/11
  Data Store Read4/12 -> Mux/12
  Data Store Read4/13 -> Mux/13
  Data Store Read4/14 -> Mux/14
  Data Store Read4/15 -> Mux/15
  Data Store Read4/16 -> Mux/16
  Data Store Read4/17 -> Mux/17
  Data Store Read4/18 -> Mux/18
  Data Store Read4/19 -> Mux/19
  Data Store Read4/20 -> Mux/20
  Saturation1/1 -> Data Type Conversion1/1
  Saturation2/1 -> Data Type Conversion2/1
  BMS_Output/1 -> Bus Selector3/1
  Bus Selector3/1 -> Balancing_Write_To_Registers/1(Bal_On_Off), Data Store Write5/1  "<BalCmd>"
  Subsystem3/1(Status_Packet2_Data_Tx) -> Bus Creator2/2  "Status_Packet2_Data_Tx"
  Subsystem1/1(Status_Packet1_Data_Tx) -> Bus Creator2/1  "Status_Packet1_Data_Tx"
  Subsystem2/1(Status_Packet4_Data_Tx) -> Bus Creator2/4  "Status_Packet4_Data_Tx"
  Bus Selector4/1 -> Data Store Write10/1  "<VCU_BMS_DATA>"
  Bus Selector4/2 -> Data Store Write11/1  "<OBC_BMS_DATA>"
  Bus Creator2/1 -> CAN_TX_RX/1
  Subsystem4/1(Status_Packet3_Data_Tx) -> Bus Creator2/3  "Status_Packet3_Data_Tx"
  CAN_TX_RX/1 -> Bus Selector4/1
  Bus Selector1/3 -> Data Store Write/3, OR/3, Cast To Double3/1  "<HighTempCharging>"
  Cast To Double4/1 -> Data Store Write16/1
  Cast To Double3/1 -> Data Store Write14/1
  Bus Selector1/4 -> Data Store Write/4, OR/4, Cast To Double2/1  "<LowTempCharging>"
  Cast To Double1/1 -> Data Store Write13/1
  Bus Selector1/2 -> Data Store Write/2, OR/2, Cast To Double4/1  "<OverCurrentCharging>"
  Cast To Double2/1 -> Data Store Write15/1
  Cast To Double/1 -> Data Store Write12/1
  Logical Operator1/1 -> RED_LED/1
  Bus Selector3/2 -> Relay/1  "<Relay>"
  BMS_Info (Duplicate)/1 -> Write EEPROM/1(BMS_Info)
  Bus Selector1/13 -> Cast To Single/1  "<BMS_State>"
  Cast To Single/1 -> Data Store Write6/1
  Cast To Double7/1 -> Data Store Write17/1
  Cast To Double6/1 -> Data Store Write9/1
  Cast To Double5/1 -> Data Store Write7/1
  Bus Selector1/5 -> OR/5, Cast To Double5/1  "<OverCurrentDischarging>"
  Bus Selector1/6 -> Cast To Double6/1, OR/6  "<HighTempDischarging>"
  Bus Selector1/7 -> Cast To Double7/1, OR/7  "<LowTempDischarging>"
  Bus Selector1/8 -> Cast To Double1/1, Data Store Write/5, OR/8  "<OverVolt>"
  Bus Selector1/9 -> Cast To Double/1, Data Store Write/6, OR/9  "<UnderVolt>"
  Bus Selector1/10 -> Data Store Write/7, OR/10  "<Charger>"
  Bus Selector1/11 -> Data Store Write/8, OR/11  "<Inverter>"
  Bus Selector1/12 -> Demux/1  "<SOC>"
